simulink model "IntelligentBinPicking"  (R2024a)
settings: Solver=FixedStepAuto  StartTime=0.0  StopTime=200  FixedStep=0.05  RelTol=1e-3
PreLoadFcn:
  | initRobotModelParam;
model workspace (MAT data in the model file):
  SL_ROS_VariableLengthArrays_MaxSizes.CommonInfo.ArrayTruncateAction = 'EmitWarning'
  SL_ROS_VariableLengthArrays_MaxSizes.MsgTypeMap = containers.Map
  SL_ROS_VariableLengthArrays_MaxSizes.MsgTypeMap.serialization.keys = {'sensor_msgs/Image', 'sensor_msgs/PointCloud2'}
  SL_ROS_VariableLengthArrays_MaxSizes.MsgTypeMap.serialization.values{1}(1).PropertyName = 'Data'
  SL_ROS_VariableLengthArrays_MaxSizes.MsgTypeMap.serialization.values{1}(1).DataType = 'uint8'
  SL_ROS_VariableLengthArrays_MaxSizes.MsgTypeMap.serialization.values{1}(1).MaxLength = 921600
  SL_ROS_VariableLengthArrays_MaxSizes.MsgTypeMap.serialization.values{1}(2).PropertyName = 'Encoding'
  SL_ROS_VariableLengthArrays_MaxSizes.MsgTypeMap.serialization.values{1}(2).DataType = 'uint8'
  SL_ROS_VariableLengthArrays_MaxSizes.MsgTypeMap.serialization.values{1}(2).MaxLength = 128
  SL_ROS_VariableLengthArrays_MaxSizes.MsgTypeMap.serialization.values{2}(1).PropertyName = 'Data'
  SL_ROS_VariableLengthArrays_MaxSizes.MsgTypeMap.serialization.values{2}(1).DataType = 'uint8'
  SL_ROS_VariableLengthArrays_MaxSizes.MsgTypeMap.serialization.values{2}(1).MaxLength = 9830400
  SL_ROS_VariableLengthArrays_MaxSizes.MsgTypeMap.serialization.values{2}(2).PropertyName = 'Fields'
  SL_ROS_VariableLengthArrays_MaxSizes.MsgTypeMap.serialization.values{2}(2).DataType = 'sensor_msgs/PointField'
  SL_ROS_VariableLengthArrays_MaxSizes.MsgTypeMap.serialization.values{2}(2).MaxLength = 16
  SL_ROS_VariableLengthArrays_MaxSizes.MsgTypeMap.serialization.uniformity = 0
  SL_ROS_VariableLengthArrays_MaxSizes.MsgTypeMap.serialization.keyType = 'char'
  SL_ROS_VariableLengthArrays_MaxSizes.MsgTypeMap.serialization.valueType = 'any'
undefined symbols (not defined in the file): binActorRotationSequenceInfo, binActorTranslationSequenceInfo, binCenterPosition, camera_rot, cameraIntrinsics, cx_camera, cy_camera, downSampleForTrajectoryWaypoints, Enable, enumCmd, f, graspRegionTranslation, gray, homePosition, IsAccValid, IsMoving, IsPosValid, isSingleDetection, IsValid, IsVelValid, JointAcc, JointCurrent, JointPos, JointTrajectory, JointVel, maxVisionObjects, Mode, motionPlannerCmdInitValue, motionPlannerResponseInitValue, NumObjects, NumPoints, objectDetectorResponseInitValue, Objects, ObjectTypesID, pickAllOrder, PickAllOrder, PickAndPlaceModes, PickSelectedObjectID, posTargetError, predictionConfidenceScore, RequestID, Reset, RGBCameraTransform, robotCommandInitValue, robotFeedbackInitValue, Sim3dSensor, Status, TargetEETranslation, targetEnv, TaskPlannerSampleTime, Time, TooltipTransform, ur5e
libraries: sim3dlib x13, robotlib x6, robotmaniplib x4, robotcorelib x1, robotsim3dlib x1, sim3dcameralib x1
(part 1 of 2)
settings Model: Creator=gjohn  LastModifiedBy=adityas
settings DebuggingCC: SubsystemReferenceDiagnosticForUnitTest=warning
settings RTWCC: GPUComputeCapability=3.5

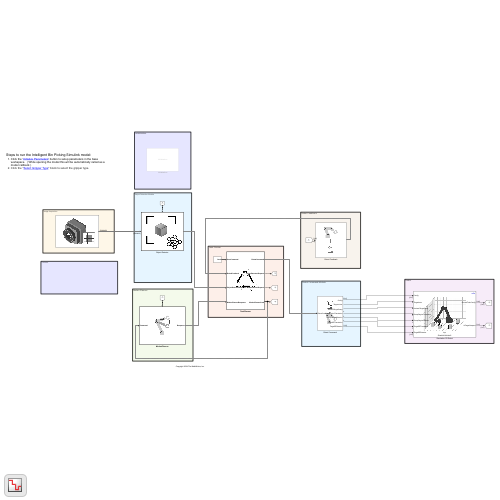
[thumbnail: Simulink's stored preview of the top-level diagram]
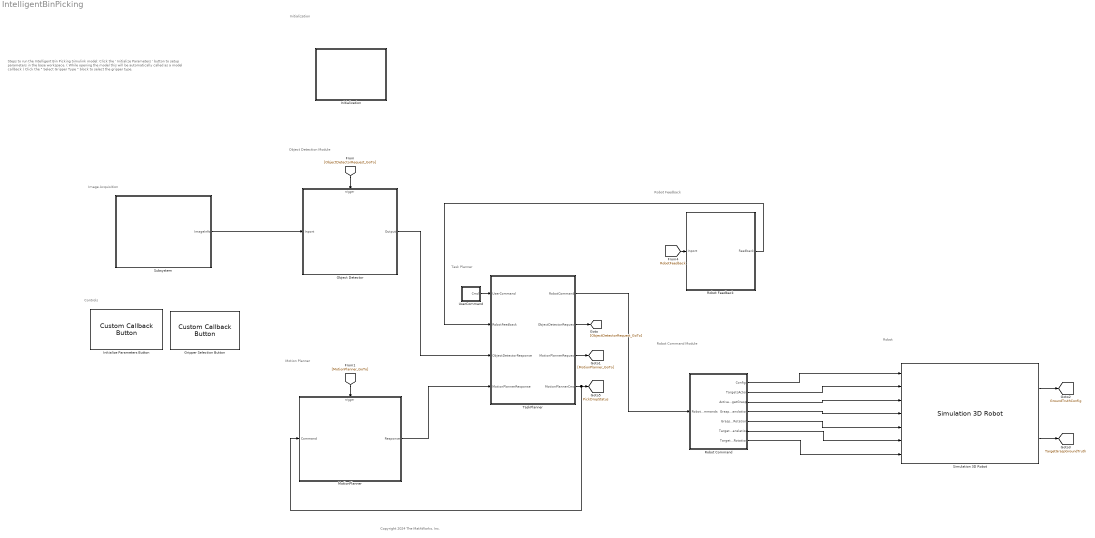
== system IntelligentBinPicking ==
  note: Steps to run the Intelligent Bin Picking Simulink model:
      | Click the ' Initialize Parameters ' button to setup parameters in the base workspace. ( While opening the model this will be automatically called as a model callback )
      | Click the " Select Gripper Type " block to select the gripper type.
  note: Task Planner
  note: Motion Planner
  note: Robot Command Module
  note: Robot Feedback
  note: Object Detection Module
  note: Controls
  note: Copyright 2024 The MathWorks, Inc.
  note: Initialization
  note: Image Acquisition
  note: Robot
  Gripper Selection Button : CustomCallbackButton  Configuration="{\"components\":[{\"name\":\"BackgroundImageComponent\",\"settings\":{\"image\":{\"size\":[0,0],\"src\":\"default\",\"srcOrientation\":\"Right\"},\"position\":[0,0,1,1]}},{\"name\":\"ButtonStateComponent\",\"settings\":{\"buttonType\":\"momentary\",\"clickFcn\":\"getGripperType;\\nfprintf('Loading Robot Model and Parameters...');\\nfprintf('\\\\n');\\nclear rbt ur5e;\\nrbt = loadrobot('universalUR5e','DataFormat','row');\\nur5e = exampleHelperAddGripper(rbt,gripperType);\\n\\ndisp(\\\"Setup complete for Robot hardware\\\");\\n\",\"onValue\":1,\"position\":[0,0,1,1],\"pressDelay\":\"500\",\"pressFcn\":\"\",\"repeatInterval\":\"0\",\"states\":[{\"horizontalAlignment\":\"center\",\"image\":{\"position\":[0,0,1,1],\"size\":[1,1],\"src\":\"default\",\"srcOrientation\":\"Right\"},\"label\":{\"color\":[0.011764705882352941,0.011764705882352941,0.011764705882352941],\"icon\":{\"size\":[0,0],\"src\":\"default\",\"srcOrientation\":\"Right\"},\"iconPlacement\":\"left\",\"opacity\":1,\"show\":true,\"text\":{\"content\":\"Select Gripper Type\",\"font\":\"Helvetica\",\"fontSize\":9.600000000000001}},\"labelOffset\":[0,0],\"verticalAlignment\":\"middle\"},{\"horizontalAlignment\":\"center\",\"image\":{\"position\":[0,0,1,1],\"size\":[1,1],\"src\":\"default\",\"srcOrientation\":\"Right\"},\"label\":{\"color\":[0.011764705882352941,0.011764705882352941,0.011764705882352941],\"icon\":{\"size\":[0,0],\"src\":\"default\",\"srcOrientation\":\"Right\"},\"iconPlacement\":\"left\",\"opacity\":1,\"show\":true,\"text\":{\"content\":\"Select Gripper Type\",\"font\":\"Helvetica\",\"fontSize\":9.600000000000001}},\"labelOffset\":[0,0],\"verticalAlignment\":\"middle\"},{\"horizontalAlignment\":\"center\",\"image\":{\"position\":[0,0,1,1],\"size\":[1,1],\"src\":\"default\",\"srcOrientation\":\"Right\"},\"label\":{\"color\":[0.011764705882352941,0.011764705882352941,0.011764705882352941],\"icon\":{\"size\":[0,0],\"src\":\"default\",\"srcOrientation\":\"Right\"},\"iconPlacement\":\"left\",\"opacity\":1,\"show\":true,\"text\":{\"content\":\"Select Gripper Type\",\"font\":\"Helvetica\",\"fontSize\":9.600000000000001}},\"labelOffset\":[0,0],\"verticalAlignment\":\"middle\"},{\"horizontalAlignment\":\"center\",\"image\":{\"position\":[0,0,1,1],\"size\":[1,1],\"src\":\"default\",\"srcOrientation\":\"Right\"},\"label\":{\"color\":[0.011764705882352941,0.011764705882352941,0.011764705882352941],\"icon\":{\"size\":[0,0],\"src\":\"default\",\"srcOrientation\":\"Right\"},\"iconPlacement\":\"left\",\"opacity\":1,\"show\":true,\"text\":{\"content\":\"Select Gripper Type\",\"font\":\"Helvetica\",\"fontSize\":9.600000000000001}},\"labelOffset\":[0,0],\"verticalAlignment\":\"middle\"}]}},{\"name\":\"ForegroundImageComponent\",\"settings\":{\"image\":{\"size\":[0,0],\"src\":\"default\",\"srcOrientation\":\"Right\"},\"isForeground\":1,\"position\":[0,0,1,1]}}],\"settings\":{\"BindingType\":\"standalone\",\"backgroundColor\":[244,244,244,1],\"backgroundOffset\":0,\"backgroundOpacity\":1,\"fixedAspectRatio\":\"off\",\"foregroundColor\":[0.01176470588,0.01176470588,0.01176470588,1],\"migratedFromLegacy\":true,\"useBackgroundColor\":true,\"variant\":\"callback\",\"version\":\"R2023a\"},\"type\":\"Button\"}"  CustomBackgroundColor="{\"color\":[0.6196078431372549,0.8392156862745098,0.9490196078431372],\"show\":true}"
  Initialization : Subsystem  Priority=0
      mask Display: disp(' Initialization ');
  Initialize Parameters Button : CustomCallbackButton  Configuration="{\"components\":[{\"name\":\"BackgroundImageComponent\",\"settings\":{\"image\":{\"size\":[0,0],\"src\":\"default\",\"srcOrientation\":\"Right\"},\"position\":[0,0,1,1]}},{\"name\":\"ButtonStateComponent\",\"settings\":{\"buttonType\":\"momentary\",\"clickFcn\":\"%%\\ninitRobotModelParam;\\ndisp('*******************************************************');\\ndisp('Parameters Initialized')\",\"onValue\":1,\"position\":[0,0,1,1],\"pressDelay\":\"500\",\"pressFcn\":\"\",\"repeatInterval\":\"0\",\"states\":[{\"horizontalAlignment\":\"center\",\"image\":{\"position\":[0,0,1,1],\"size\":[1,1],\"src\":\"default\",\"srcOrientation\":\"Right\"},\"label\":{\"color\":[0,0,0],\"icon\":{\"size\":[0,0],\"src\":\"default\",\"srcOrientation\":\"Right\"},\"iconPlacement\":\"left\",\"opacity\":1,\"show\":true,\"text\":{\"content\":\"Initialize Parameters\",\"font\":\"Helvetica\",\"fontSize\":3.823752}},\"labelOffset\":[0,0],\"verticalAlignment\":\"middle\"},{\"horizontalAlignment\":\"center\",\"image\":{\"position\":[0,0,1,1],\"size\":[1,1],\"src\":\"default\",\"srcOrientation\":\"Right\"},\"label\":{\"color\":[0.01176470588,0.01176470588,0.01176470588,1],\"icon\":{\"size\":[0,0],\"src\":\"default\",\"srcOrientation\":\"Right\"},\"iconPlacement\":\"left\",\"opacity\":1,\"show\":true,\"text\":{\"content\":\"Initialize Parameters\",\"font\":\"Helvetica\",\"fontSize\":3.823752}},\"labelOffset\":[0,0],\"verticalAlignment\":\"middle\"},{\"horizontalAlignment\":\"center\",\"image\":{\"position\":[0,0,1,1],\"size\":[1,1],\"src\":\"default\",\"srcOrientation\":\"Right\"},\"label\":{\"color\":[0.01176470588,0.01176470588,0.01176470588,1],\"icon\":{\"size\":[0,0],\"src\":\"default\",\"srcOrientation\":\"Right\"},\"iconPlacement\":\"left\",\"opacity\":1,\"show\":true,\"text\":{\"content\":\"Initialize Parameters\",\"font\":\"Helvetica\",\"fontSize\":3.823752}},\"labelOffset\":[0,0],\"verticalAlignment\":\"middle\"},{\"horizontalAlignment\":\"center\",\"image\":{\"position\":[0,0,1,1],\"size\":[1,1],\"src\":\"default\",\"srcOrientation\":\"Right\"},\"label\":{\"color\":[0.01176470588,0.01176470588,0.01176470588,1],\"icon\":{\"size\":[0,0],\"src\":\"default\",\"srcOrientation\":\"Right\"},\"iconPlacement\":\"left\",\"opacity\":1,\"show\":true,\"text\":{\"content\":\"Initialize Parameters\",\"font\":\"Helvetica\",\"fontSize\":3.823752}},\"labelOffset\":[0,0],\"verticalAlignment\":\"middle\"}]}},{\"name\":\"ForegroundImageComponent\",\"settings\":{\"image\":{\"size\":[0,0],\"src\":\"default\",\"srcOrientation\":\"Right\"},\"isForeground\":1,\"position\":[0,0,1,1]}}],\"settings\":{\"BindingType\":\"standalone\",\"backgroundColor\":[244,244,244,1],\"backgroundOffset\":0,\"backgroundOpacity\":1,\"fixedAspectRatio\":\"off\",\"foregroundColor\":[0.01176470588,0.01176470588,0.01176470588,1],\"migratedFromLegacy\":true,\"useBackgroundColor\":true,\"variant\":\"callback\",\"version\":\"R2023a\"},\"type\":\"Button\"}"  CustomBackgroundColor="{\"color\":[0.6196078431372549,0.8392156862745098,0.9490196078431372],\"show\":true}"
  MotionPlanner : Subsystem
      mask Display: image('$imagefile'); % Use "Edit Image" on toolstrip to change.
  Object Detector : Subsystem  TreatAsAtomicUnit=on
      mask Display: image('$imagefile'); % Use "Edit Image" on toolstrip to change.
  Robot Command : Subsystem
      mask Display: image('SLToRobotComm.png');
  Robot Feedback : Subsystem
      mask Display: image('$imagefile'); % Use "Edit Image" on toolstrip to change.
  Simulation 3D Robot : robotsim3dlib/Simulation 3D Robot  actorInputType=RigidBodyTree Object  RigidBodyTree=ur5e  ActorName=SimulinkVehicle2  existActorChekBox=off  initialTrans=robotInitialBaseTranslation  initialRot=robotInitialBaseRotation  initialConfig=homePosition  EndEffector=tcp  eeOffsetInpChekBox=on  eeTargetTrans=[0 0 0.015 ]  eeTargetRot=[ 0 0 0 ]  enableRegionGraspChekBox=on  regionGraspInpChekBox=on  eeTargTransDiff=[ 0.2 0.2 0.2 ]  eeTargRotDiff=[ 0 0 0 ]  inpConfEnbVal=on  inpGraspEnbVal=on  inpTransEnbVal=off  outConfEnbVal=on  outGraspEnbVal=on  outTransEnbVal=off  SampleTime=-1  ActorType=SimulinkVehicle  ID=2  aMode=6  ActorTag=SimulinkVehicle2  Mesh=RigidBodyTree
  Subsystem : Subsystem
      mask Display:
      | IconInfoM = sim3dblkssharedicon('sim3dblkscamerasensor', gcb, 'DrawCommands');
      | image(IconInfoM.image);
  TaskPlanner : Subsystem  TreatAsAtomicUnit=on  SystemSampleTime=TaskPlannerSampleTime
      mask Display: image('$imagefile'); % Use "Edit Image" on toolstrip to change.
  UserCommand : Subsystem
  tag scope: GroundTruthConfig=global, PickDropStatus=global, TargetGraspGroundTruth=global
  wires:
  UserCommand/1(Cmd) -> TaskPlanner/1(UserCommand)
  TaskPlanner/2(ObjectDetectorRequest) -> [ObjectDetectorRequest_GoTo]
  [ObjectDetectorRequest_GoTo] -> Object Detector/Trigger
  TaskPlanner/3(MotionPlannerRequest) -> [MotionPlanner_GoTo]
  [MotionPlanner_GoTo] -> MotionPlanner/Trigger
  TaskPlanner/4(MotionPlannerCmd) -> [PickDropStatus], MotionPlanner/1(Command)
  MotionPlanner/1(Response) -> TaskPlanner/4(MotionPlannerResponse)
  Object Detector/1(Output) -> TaskPlanner/3(ObjectDetectorResponse)
  Robot Feedback/1(Feedback) -> TaskPlanner/2(RobotFeedback)
  Simulation 3D Robot/1 -> [GroundTruthConfig]
  Simulation 3D Robot/2 -> [TargetGraspGroundTruth]
  [RobotFeedback] -> Robot Feedback/1(Inport)
  Subsystem/1(ImageInfo) -> Object Detector/1(Inport)
  TaskPlanner/1(RobotCommand) -> Robot Command/1(RobotCommands)
  Robot Command/1(Config) -> Simulation 3D Robot/1
  Robot Command/2(TargetcActor) -> Simulation 3D Robot/2
  Robot Command/3(ActivateTargetGrasp) -> Simulation 3D Robot/3
  Robot Command/4(GraspRegionTranslation) -> Simulation 3D Robot/4
  Robot Command/5(GraspRegionRotation) -> Simulation 3D Robot/5
  Robot Command/6(TargetEETranslation) -> Simulation 3D Robot/6
  Robot Command/7(TargetEERotation) -> Simulation 3D Robot/7

== system IntelligentBinPicking/Initialization ==
  Sim3d Scene Generation : Subsystem
      mask Display:
      | IconInfo = sim3dblkssharedicon('sim3dblksgenericactor',gcb,'DrawCommands');
      | image(IconInfo.image);
  Simulation 3D Scene Configuration : sim3dlib/Simulation 3D Scene Configuration  Priority=0  ProjectFormat=Default Scenes  SceneDesc=Empty scene  ProjectName=S:\41\adityas.BR2024ad.j2628055.GeckIBP\matlab\toolbox\shared\sim3d_projects\automotive_project_windows\UE\WindowsNoEditor\VehicleSimulation.exe  ScenePath=/Game/Maps/HwStrght  EnableOpenDRIVE=off  vehTagList={'BackPlane';'CelingPlane';'Custom';'FrontPlane';'GroundPlane';'LeftPlane';'RightPlane';'Scene Origin';'Sim3dActor1';'Sim3dActor2';'Sim3dActor3';'Sim3dActor4';'Sim3dActor5';'SimulinkVehicle2';'TableStand'}  vehTag=Custom  FreeCameraInitialTranslation=[0.25 1.5 1.0]  FreeCameraDefaultInitialTranslation=[-6, 0, 2]  FreeCameraInitialRotation=[-30, 0, -100]  FreeCameraDefaultInitialRotation=[0, -15, 0]  OpVisEn=off  Ts=0.05  EnableWindow=on  EnableRemoteAccess=off  EnableWeather=on  SunAzimuth=180  SunAltitude=90  EnableGeospatialSun=off  Latitude=0  Longitude=0  Date=2023-01-01  Time=10:30:00  GeoTimeZone=-5.0  SunDaylightSaving=off  wind=-6.0  clouds=0  EnableVolumetricClouds=off  CloudCoverage=50  CloudAltitude=5  fog=0  rain=0  RaindropsEffect=off  SnowDensity=0  EnableGeospatial=off  UseTrueOrigin=off  OriginHeight=200  OriginLatitude=40.744652  OriginLongitude=-73.988864  MapStyle=Aerial  AdditionalAssetIDs=[]  UseAdvancedSunSky=off  SolarTime=11  TimeZone=-5  Day=21  Month=9  Year=2022  UseDaylightSavingTime=on  DSTStartDay=10  DSTStartMonth=3  DSTEndDay=3  DSTEndMonth=11  DSTSwitchHour=2  sensorTag=MainCamera1  sensorId=1  sensorName=MainCamera1  mountLoc=Origin  offsetFlag=off  tmountOffset=[0, 0, 0]  rmountOffset=[0, 0, 0]  HorizontalResolution=1280  VerticalResolution=720  HorizontalFOV=60  mountPoint=[0 0 0]  mountOrientation=[0 0 0]  aMode=5  ID=1  GeoTrigger=Inactive
      settings: LibrarySourceBlock=sl3dlib/Simulation 3D/Simulation 3D Scene Configuration

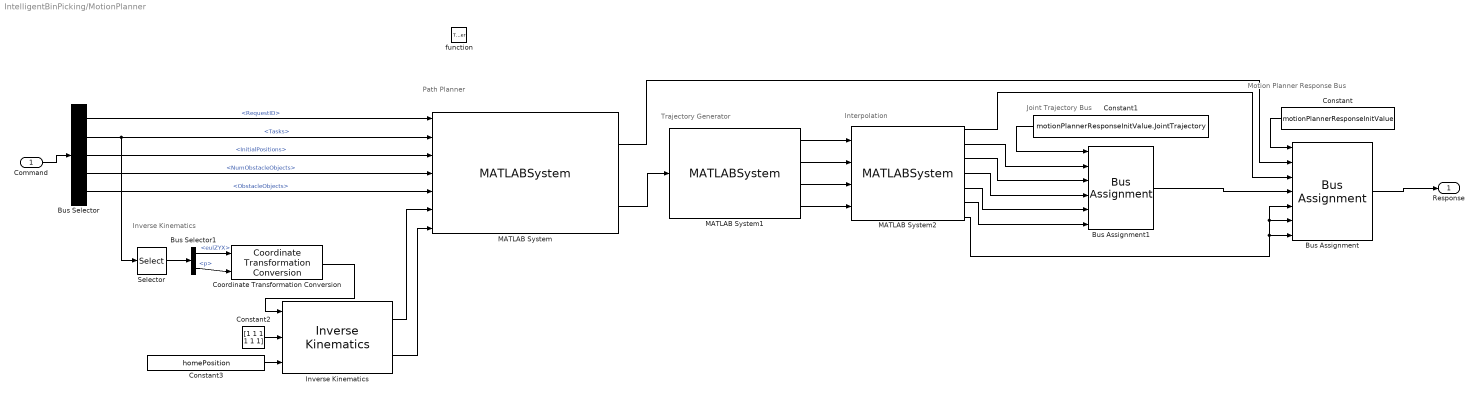
== system IntelligentBinPicking/MotionPlanner ==
  note: Interpolation
  note: Trajectory Generator
  note: Path Planner
  note: Inverse Kinematics
  note: Joint Trajectory Bus
  note: Motion Planner Response Bus
  Command : Inport  OutDataTypeStr=Bus: BUS_motion_planner_cmd
  function : TriggerPort  TriggerType=function-call  VariantControl=Variant  PortDimensions=1
  Bus Assignment : BusAssignment  AssignedSignals=RequestID,Status,JointTrajectory,IsPosValid,IsVelValid,IsAccValid
  Bus Assignment1 : BusAssignment  AssignedSignals=NumPoints,Time,JointPos,JointVel,JointAcc
  Bus Selector : BusSelector  OutputSignals=RequestID,Tasks,InitialPositions,NumObstacleObjects,ObstacleObjects
  Bus Selector1 : BusSelector  OutputSignals=eulZYX,p
  Constant : Constant  Value=motionPlannerResponseInitValue  OutDataTypeStr=Bus: BUS_motion_planner_response
  Constant1 : Constant  Value=motionPlannerResponseInitValue.JointTrajectory  OutDataTypeStr=Bus: BUS_joint_trajectory
  Constant2 : Constant  Value=[1 1 1 1 1 1]
  Constant3 : Constant  Value=homePosition
  Coordinate Transformation Conversion : robotcorelib/Coordinate Transformation Conversion  InputRepresentation=Euler Angles  InputEulerSequence=ZYX  ShowTrVecInputPort=on  OutputRepresentation=Homogeneous Transformation  OutputEulerSequence=ZYX  ShowTrVecOutputPort=on  SimulateUsing=Code generation
  Inverse Kinematics : robotmaniplib/Inverse Kinematics  RigidBodyTree=ur5e  EndEffector=tcp  ShowInfo=on  SolverName=BFGS Gradient Projection  EnforceJointLimits=on  MaxIterations=1500  MaxTime=10  GradientTolerance=1e-7  SolutionTolerance=1e-6  StepTolerance=1e-14  ErrorChangeTolerance=1e-12  UseErrorDamping=on  DampingBias=0.0025  SimulateUsing=Code generation
  MATLAB System : MATLABSystem  System=MotionPlannerCHOMP  BinLength=binLength  BinHeight=binHeight  BinWidth=binWidth  BinRotation=binRotation  BinCenterPosition=binCenterPosition  HomePosition=retractHomePosition  Target=targetEnv  GripperType=gripperType  IsMEXed=off  SimulateUsing=Interpreted execution
      mask Type: MotionPlannerCHOMP
      mask Display:
      | disp('MotionPlannerCHOMP');
      | port_label('input',1,'requestID');
      | port_label('input',2,'tasks');
      | port_label('input',3,'q0');
      | port_label('input',4,'numObstacles');
      | port_label('input',5,'obstacles');
      | port_label('input',6,'configSoln');
      | port_label('input',7,'configSolnInfo');
      | port_label('output',1,'reqID');
      | port_label('output',2,'path');
  MATLAB System1 : MATLABSystem  System=Contopptraj  VelocityLimits=vellimits  AccelLimits=accellimits  NumSamples=50  SimulateUsing=Interpreted execution
      mask Type: Contopptraj
      mask Display:
      | disp('Contopptraj');
      | port_label('input',1,'planPath');
      | port_label('output',1,'q');
      | port_label('output',2,'qd');
      | port_label('output',3,'qdd');
      | port_label('output',4,'t');
  MATLAB System2 : MATLABSystem  System=Interpolation  trajectorySampleTime=1 / 400  MaxNumPoints=maxNumPoints  SimulateUsing=Code generation
      mask Type: Interpolation
      mask Display:
      | disp('Interpolation');
      | port_label('input',1,'q');
      | port_label('input',2,'qd');
      | port_label('input',3,'qdd');
      | port_label('input',4,'t');
      | port_label('output',1,'status');
      | port_label('output',2,'numPoints');
      | port_label('output',3,'time');
      | port_label('output',4,'jointPos');
      | port_label('output',5,'jointVel');
      | port_label('output',6,'jointAcc');
      | port_label('output',7,'isValid');
  Selector : Selector  InputPortWidth=20  IndexOptions=Index vector (dialog)  Indices=1  OutputSizes=1
  Response : Outport  OutDataTypeStr=Bus: BUS_motion_planner_response  InitialOutput=motionPlannerResponseInitValue  VectorParamsAs1DForOutWhenUnconnected=off
  wires:
  Bus Selector1/2 -> Coordinate Transformation Conversion/2  "<p>"
  Bus Selector/3 -> MATLAB System/3  "<InitialPositions>"
  Constant2/1 -> Inverse Kinematics/2
  Selector/1 -> Bus Selector1/1
  Bus Selector/2 -> MATLAB System/2, Selector/1  "<Tasks>"
  Coordinate Transformation Conversion/1 -> Inverse Kinematics/1
  Inverse Kinematics/1 -> MATLAB System/6
  Bus Selector1/1 -> Coordinate Transformation Conversion/1  "<eulZYX>"
  Command/1 -> Bus Selector/1
  Bus Selector/1 -> MATLAB System/1  "<RequestID>"
  MATLAB System2/1 -> Bus Assignment/3
  MATLAB System/1 -> Bus Assignment/2
  MATLAB System2/3 -> Bus Assignment1/3
  MATLAB System2/5 -> Bus Assignment1/5
  MATLAB System2/6 -> Bus Assignment1/6
  Bus Assignment/1 -> Response/1
  Constant1/1 -> Bus Assignment1/1
  MATLAB System2/4 -> Bus Assignment1/4
  MATLAB System2/2 -> Bus Assignment1/2
  Constant/1 -> Bus Assignment/1
  Bus Assignment1/1 -> Bus Assignment/4
  MATLAB System2/7 -> Bus Assignment/5, Bus Assignment/6, Bus Assignment/7
  Bus Selector/4 -> MATLAB System/4  "<NumObstacleObjects>"
  Bus Selector/5 -> MATLAB System/5  "<ObstacleObjects>"
  MATLAB System1/1 -> MATLAB System2/1
  MATLAB System1/2 -> MATLAB System2/2
  MATLAB System1/3 -> MATLAB System2/3
  MATLAB System1/4 -> MATLAB System2/4
  MATLAB System/2 -> MATLAB System1/1
  Inverse Kinematics/2 -> MATLAB System/7
  Constant3/1 -> Inverse Kinematics/3

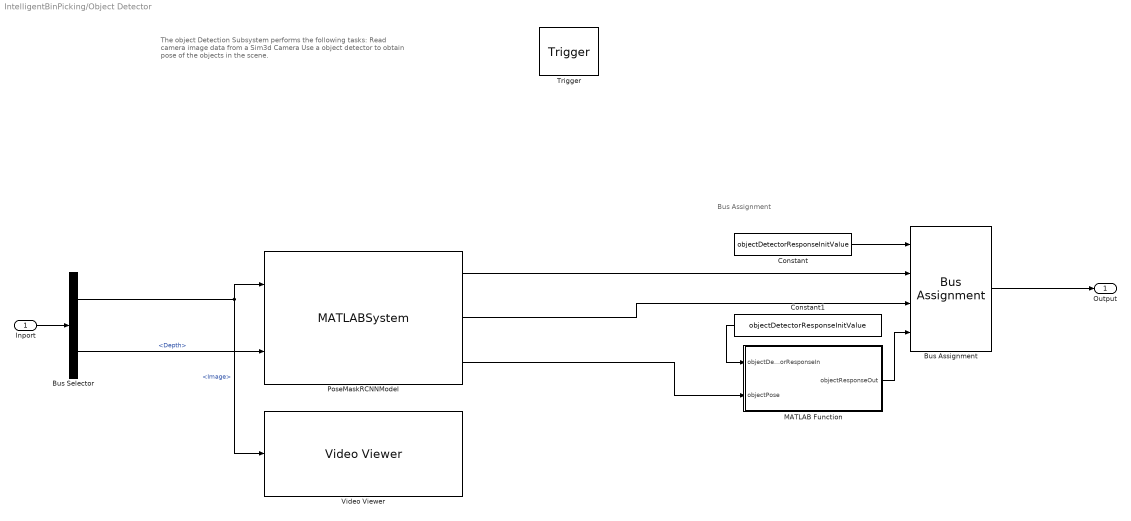
== system IntelligentBinPicking/Object Detector ==
  note: Bus Assignment
  note: The object Detection Subsystem performs the following tasks:
      | Read camera image data from a Sim3d Camera
      | Use a object detector to obtain pose of the objects in the scene.
  Inport : Inport
  Trigger : TriggerPort  TriggerType=function-call  VariantControl=(inherit)
  Bus Assignment : BusAssignment  AssignedSignals=Status,NumObjects,Objects
  Bus Selector : BusSelector  OutputSignals=Image,Depth
  Constant : Constant  Value=objectDetectorResponseInitValue  OutDataTypeStr=Bus: BUS_object_detector_response
  Constant1 : Constant  Value=objectDetectorResponseInitValue  OutDataTypeStr=Bus: BUS_object_detector_response
  MATLAB Function : MATLAB Function  TreatAsAtomicUnit=on
  PoseMaskRCNNModel : MATLABSystem  System=PoseMaskRCNNModel  NetName=resnet50-pvc-parts  MaxDepth=maxDepth  MaxBinDistance=maxBinDistance  BinOrientation=binOrientation  TargetBinaryMask=targetAreaMask  CameraLoc=camera_loc  CameraRot=camera_rot  Intrinsics="cameraIntrinsics( [ 750, 750 ], [ 640, 360 ], [ 720, 1280 ], \"RadialDistortion\", [ 0, 0 ], \"TangentialDistortion\", [ 0, 0 ], \"Skew\", 0 )"  MaxObjectDectection=maxObjectDetection  Threshold=predictionConfidenceScore  RobotOffset=robotInitialBaseTranslation  ExecutionEnvironment=gpu
      mask Type: PoseMaskRCNNModel
      mask Display:
      | disp('PoseMaskRCNNModel');
      | port_label('input',1,'imRGB');
      | port_label('input',2,'imDepth');
      | port_label('output',1,'status');
      | port_label('output',2,'numObjects');
      | port_label('output',3,'objectPose');
  Video Viewer : VideoViewer  colormapValue=gray(256)  FigPos=[345 622 589.333333333333 526]
  Output : Outport
  wires:
  Constant/1 -> Bus Assignment/1
  PoseMaskRCNNModel/1 -> Bus Assignment/2
  PoseMaskRCNNModel/2 -> Bus Assignment/3
  Bus Assignment/1 -> Output/1
  Constant1/1 -> MATLAB Function/1(objectDetectorResponseIn)
  PoseMaskRCNNModel/3 -> MATLAB Function/2(objectPose)
  MATLAB Function/1(objectResponseOut) -> Bus Assignment/4
  Bus Selector/1 -> PoseMaskRCNNModel/1, Video Viewer/1  "<Image>"
  Bus Selector/2 -> PoseMaskRCNNModel/2  "<Depth>"
  Inport/1 -> Bus Selector/1

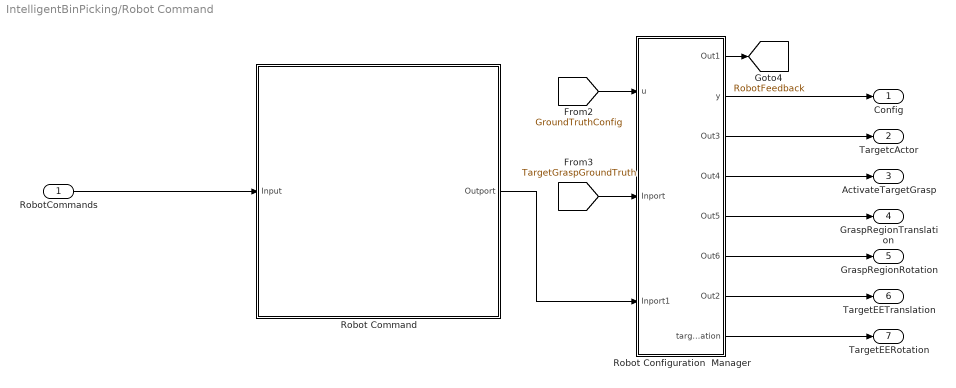
== system IntelligentBinPicking/Robot Command ==
  RobotCommands : Inport
  Robot Command : Subsystem
      mask Display: image('SLToRobotComm.png'); % Use "Edit Image" on toolstrip to change.
  Robot Configuration  Manager : Subsystem  mask{RobotRigidTree=ur5e, ActorTranslationConfig=binActorTranslationSequenceInfo, ActorRotationConfig=binActorRotationSequenceInfo, HomePosition=homePosition, SamplesToConsider=downSampleForTrajectoryWaypoints, GraspRegionTranslation=graspRegionTranslation, TargetEETranslation=TargetEETranslation}
      mask prompts: RobotRigidTree "Robot rigid tree"; ActorTranslationConfig "Actor translation config"; ActorRotationConfig "Actor rotation config"; HomePosition "Robot home position"; SamplesToConsider "Samples to consider"; GraspRegionTranslation "Grasp region translation"; TargetEETranslation "Target-EE Translation"
      mask Display: disp('Config Manager');
  Config : Outport
  TargetcActor : Outport  Port=2
  ActivateTargetGrasp : Outport  Port=3
  GraspRegionTranslation : Outport  Port=4
  GraspRegionRotation : Outport  Port=5
  TargetEETranslation : Outport  Port=6
  TargetEERotation : Outport  Port=7
  tag scope: RobotFeedback=global
  wires:
  Robot Configuration  Manager/1(Out1) -> [RobotFeedback]
  Robot Configuration  Manager/2(y) -> Config/1
  [TargetGraspGroundTruth] -> Robot Configuration  Manager/2(Inport)
  [GroundTruthConfig] -> Robot Configuration  Manager/1(u)
  Robot Configuration  Manager/4(Out4) -> ActivateTargetGrasp/1
  Robot Command/1(Outport) -> Robot Configuration  Manager/3(Inport1)
  Robot Configuration  Manager/5(Out5) -> GraspRegionTranslation/1
  Robot Configuration  Manager/3(Out3) -> TargetcActor/1
  RobotCommands/1 -> Robot Command/1(Input)
  Robot Configuration  Manager/6(Out6) -> GraspRegionRotation/1
  Robot Configuration  Manager/7(Out2) -> TargetEETranslation/1
  Robot Configuration  Manager/8(targetBinActorOrientation) -> TargetEERotation/1

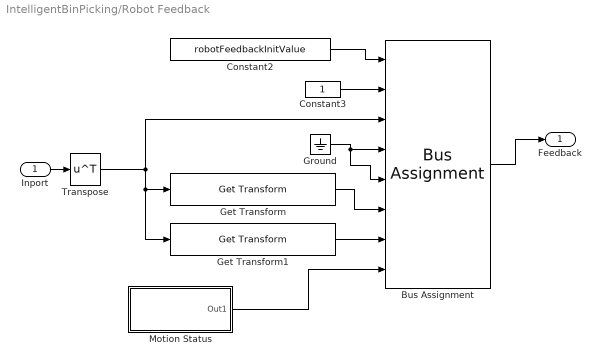
== system IntelligentBinPicking/Robot Feedback ==
  Inport : Inport
  Bus Assignment : BusAssignment  AssignedSignals=IsValid,JointPos,JointVel,JointCurrent,TooltipTransform,RGBCameraTransform,IsMoving
  Constant2 : Constant  Value=robotFeedbackInitValue  OutDataTypeStr=Bus: BUS_robot_feedback
  Constant3 : Constant  OutDataTypeStr=boolean
  Get Transform : robotmaniplib/Get Transform  RigidBodyTree=ur5e  SourceBody=tcp  TargetBody=base_link  SimulateUsing=Interpreted execution
  Get Transform1 : robotmaniplib/Get Transform  RigidBodyTree=ur5e  SourceBody=base_link  TargetBody=base_link  SimulateUsing=Interpreted execution
  Ground : Ground
  Motion Status : Subsystem  Variant=on
  Transpose : Math  Operator=transpose
  Feedback : Outport  OutDataTypeStr=Bus: BUS_robot_feedback  VectorParamsAs1DForOutWhenUnconnected=off
  wires:
  Get Transform1/1 -> Bus Assignment/7
  Constant2/1 -> Bus Assignment/1
  Bus Assignment/1 -> Feedback/1
  Ground/1 -> Bus Assignment/5, Bus Assignment/4
  Get Transform/1 -> Bus Assignment/6
  Constant3/1 -> Bus Assignment/2
  Motion Status/1(Out1) -> Bus Assignment/8
  Transpose/1 -> Bus Assignment/3, Get Transform1/1, Get Transform/1
  Inport/1 -> Transpose/1

== system IntelligentBinPicking/Subsystem ==
  Bus Creator : BusCreator  Inputs=2
  Simulation 3D Camera1 : sim3dcameralib/Simulation 3D Camera  Priority=1  sensorTag=Sim3dSensor�  sensorId=4  sensorName=Sim3dSensor�  vehTagList={'BackPlane';'CelingPlane';'FrontPlane';'GroundPlane';'LeftPlane';'RightPlane';'Scene Origin';'Sim3dActor1';'Sim3dActor2';'SimulinkVehicle2';'TableStand'}  vehTag=Scene Origin  mountLoc=Origin  offsetFlag=on  tmountOffset=camera_loc  extTmount=off  rmountOffset=rad2deg(camera_rot)  extRmount=off  FocalLength=[f, f]  OpticalCenter=[cx_camera, cy_camera]  ImageSize=imageSize  RadialDistortion=[0, 0]  TangentialDistortion=[0, 0]  SensorSkew=0  DepthOutportEnabled=on  SemanticOutportEnabled=off  TransformOutportEnabled=off  SampleTime=-1  mountPoint=[0.48 0 1.15]  mountOrientation=[90 -90 -90]  aMode=3  ID=4
      settings: LibrarySourceBlock=drivingsim3d/Simulation 3D Camera
  ImageInfo : Outport
  wires:
  Simulation 3D Camera1/1 -> Bus Creator/1  "Image"
  Simulation 3D Camera1/2 -> Bus Creator/2  "Depth"
  Bus Creator/1 -> ImageInfo/1

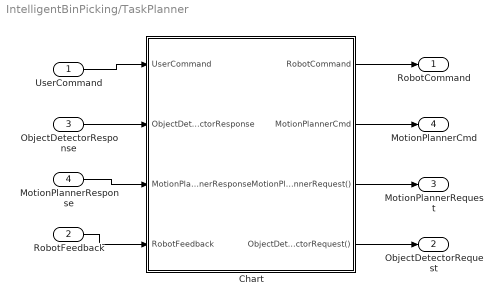
== system IntelligentBinPicking/TaskPlanner ==
  UserCommand : Inport
  RobotFeedback : Inport  Port=2  OutDataTypeStr=Bus: BUS_robot_feedback
  ObjectDetectorResponse : Inport  Port=3  OutDataTypeStr=Bus: BUS_object_detector_response
  MotionPlannerResponse : Inport  Port=4
  Chart : Stateflow chart  TreatAsAtomicUnit=on
  RobotCommand : Outport  OutDataTypeStr=Bus: BUS_robot_command  VectorParamsAs1DForOutWhenUnconnected=off
  ObjectDetectorRequest : Outport  Port=2  VectorParamsAs1DForOutWhenUnconnected=off
  MotionPlannerRequest : Outport  Port=3  VectorParamsAs1DForOutWhenUnconnected=off
  MotionPlannerCmd : Outport  Port=4  OutDataTypeStr=Bus: BUS_motion_planner_cmd  VectorParamsAs1DForOutWhenUnconnected=off
  wires:
  Chart/3(MotionPlannerRequest()) -> MotionPlannerRequest/1
  Chart/2(MotionPlannerCmd) -> MotionPlannerCmd/1
  MotionPlannerResponse/1 -> Chart/3(MotionPlannerResponse)
  Chart/4(ObjectDetectorRequest()) -> ObjectDetectorRequest/1
  ObjectDetectorResponse/1 -> Chart/2(ObjectDetectorResponse)
  Chart/1(RobotCommand) -> RobotCommand/1
  UserCommand/1 -> Chart/1(UserCommand)
  RobotFeedback/1 -> Chart/4(RobotFeedback)

== system IntelligentBinPicking/UserCommand ==
  Bus Assignment : BusAssignment  AssignedSignals=Mode,PickSelectedObjectID,PickAllOrder,Enable,Reset
  Bus_0 : Constant  Value=0  OutDataTypeStr=Bus: BUS_user_command
  Enable : Constant  OutDataTypeStr=boolean
  Mode : Constant  Value=PickAndPlaceModes.PickAll  OutDataTypeStr=Enum: PickAndPlaceModes
  ObjectToPick : Constant  Value=ObjectTypesID.X
  PickAllOrder : Constant  Value=pickAllOrder
  Reset : Constant  Value=0  OutDataTypeStr=boolean
  Cmd : Outport  OutDataTypeStr=Bus: BUS_user_command  VectorParamsAs1DForOutWhenUnconnected=off
  wires:
  Bus_0/1 -> Bus Assignment/1
  Bus Assignment/1 -> Cmd/1
  ObjectToPick/1 -> Bus Assignment/3
  Enable/1 -> Bus Assignment/5
  Reset/1 -> Bus Assignment/6
  Mode/1 -> Bus Assignment/2
  PickAllOrder/1 -> Bus Assignment/4

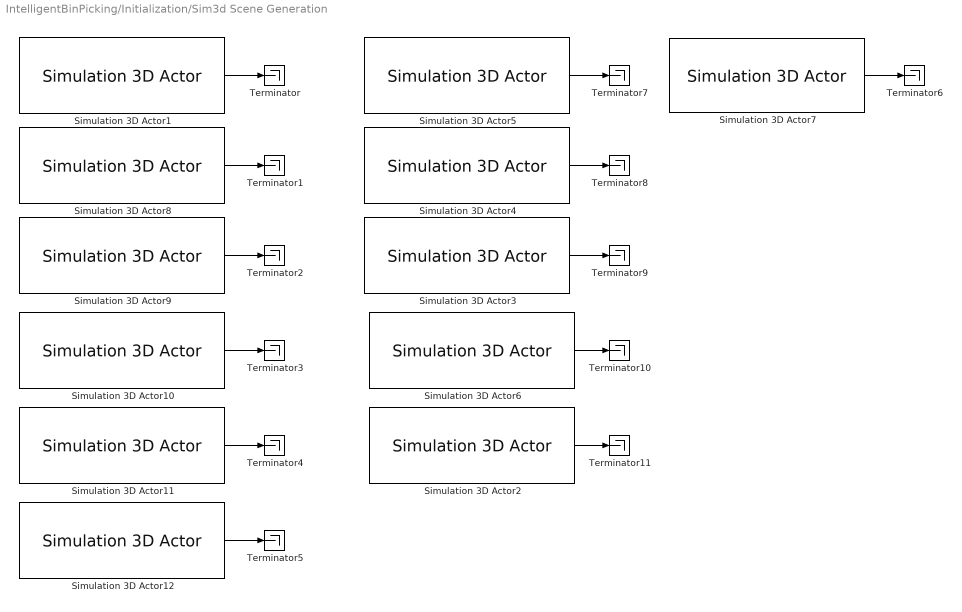
== system IntelligentBinPicking/Initialization/Sim3d Scene Generation ==
  Simulation 3D Actor1 : sim3dlib/Simulation 3D Actor  ActorName=GroundPlane  ParentName=Scene Origin  Operation=Create at setup  InitScriptText=|  SampleTime=-1  Translation=single([0 0 0])  Rotation=single([0 0 0])  Scale=single([1 1 1])  aMode=5  ActorTag=GroundPlane  ActorType=Sim3dActor  ID=C
      | Actor.createShape('box', [3 3 0.05]);
      | Actor.Color=[0.1 0.1 0.1];
      | Actor.Translation=[0 0 0];
      | Actor.Mobility=sim3d.utils.MobilityTypes.Movable;
      | Actor.ConstantAttributes=false;
      settings: LibrarySourceBlock=sl3dlib/Simulation 3D/Simulation 3D Actor
  Simulation 3D Actor10 : sim3dlib/Simulation 3D Actor  ActorName=Sim3dActor3  ParentName=Scene Origin  Operation=Create at setup  InitScriptText=|  SampleTime=-1  Translation=single([0 0 0])  Rotation=single([0 0 0])  Scale=single([1 1 1])  aMode=5  ActorTag=Sim3dActor3  ActorType=Sim3dActor  ID=3
      | %Guider
      | Actor.createShape('box', [0.0050, 0.2000, 0.0050]);
      | Actor.Translation=[0.05 -0.49 0.58];
      | Actor.Rotation=[0 pi/2 pi/2];
      | Actor.Shadows = 0;
      | Actor.Metallic = 0.70;
      | Actor.Color =[0.6824,0.4706,0.4667];
      | Actor.PreciseContacts=true;
      | Actor.Shininess=0.30;
      | Actor.Mobility=sim3d.utils.MobilityTypes.Movable;
      | Actor.ConstantAttributes=false;
      | Actor.Hidden=true;
      settings: LibrarySourceBlock=sl3dlib/Simulation 3D/Simulation 3D Actor
  Simulation 3D Actor11 : sim3dlib/Simulation 3D Actor  ActorName=Sim3dActor4  ParentName=Scene Origin  Operation=Create at setup  InitScriptText=|  SampleTime=-1  Translation=single([0 0 0])  Rotation=single([0 0 0])  Scale=single([1 1 1])  aMode=5  ActorTag=Sim3dActor4  ActorType=Sim3dActor  ID=4
      | %Guider
      | Actor.createShape('box', [0.0050, 0.2000, 0.0050]);
      | Actor.Translation=[0.05 -0.9 0.58];
      | Actor.Rotation=[0 pi/2 pi/2];
      | Actor.Shadows = 0;
      | Actor.Metallic = 0.70;
      | Actor.Color =[0.6824,0.4706,0.4667];
      | Actor.PreciseContacts=true;
      | Actor.Shininess=0.30;
      | Actor.Mobility=sim3d.utils.MobilityTypes.Movable;
      | Actor.ConstantAttributes=false;
      | Actor.Hidden=true;
      settings: LibrarySourceBlock=sl3dlib/Simulation 3D/Simulation 3D Actor
  Simulation 3D Actor12 : sim3dlib/Simulation 3D Actor  ActorName=Sim3dActor5  ParentName=Scene Origin  Operation=Create at setup  InitScriptText=|  SampleTime=-1  Translation=single([0 0 0])  Rotation=single([0 0 0])  Scale=single([1 1 1])  aMode=5  ActorTag=Sim3dActor5  ActorType=Sim3dActor  ID=5
      | %Guider
      | Actor.createShape('box', [0.0050, 0.2000, 0.0050]);
      | Actor.Translation=[0.05 0.5 0.56];
      | Actor.Rotation=[0 pi/2 pi/2];
      | Actor.Shadows = 0;
      | Actor.Metallic = 0.70;
      | Actor.Color =[0.6824,0.4706,0.4667];
      | Actor.PreciseContacts=true;
      | Actor.Shininess=0.30;
      | Actor.Mobility=sim3d.utils.MobilityTypes.Movable;
      | Actor.ConstantAttributes=false;
      | Actor.Hidden=true;
      settings: LibrarySourceBlock=sl3dlib/Simulation 3D/Simulation 3D Actor
  Simulation 3D Actor2 : sim3dlib/Simulation 3D Actor  ActorName=RightPlane  ParentName=Scene Origin  Operation=Create at setup  InitScriptText=|  SampleTime=-1  Translation=single([0 0 0])  Rotation=single([0 0 0])  Scale=single([1 1 1])  aMode=5  ActorTag=RightPlane  ActorType=Sim3dActor  ID=C
      | Actor.createShape('box', [3 3 0.05]);
      | Actor.Color=[0.1 0.1 0.1];
      | Actor.Translation=[0 1.5 0.924];
      | Actor.Rotation=[pi/2 0 0];
      | Actor.Scale=[1,0.635,1];
      | Actor.Mobility=sim3d.utils.MobilityTypes.Movable;
      | Actor.ConstantAttributes=false;
      | Actor.Collisions=false;
      settings: LibrarySourceBlock=sl3dlib/Simulation 3D/Simulation 3D Actor
  Simulation 3D Actor3 : sim3dlib/Simulation 3D Actor  ActorName=FrontPlane  ParentName=Scene Origin  Operation=Create at setup  InitScriptText=|  SampleTime=-1  Translation=single([0 0 0])  Rotation=single([0 0 0])  Scale=single([1 1 1])  aMode=5  ActorTag=FrontPlane  ActorType=Sim3dActor  ID=C
      | Actor.createShape('box', [3 3 0.05]);
      | Actor.Color=[0.1 0.1 0.1];
      | Actor.Translation=[-1.5 0 0.924];
      | Actor.Scale=[0.635,1,1];
      | Actor.Rotation=[0 pi/2 0];
      | Actor.Mobility=sim3d.utils.MobilityTypes.Movable;
      | Actor.ConstantAttributes=false;
      | Actor.Collisions=false;
      settings: LibrarySourceBlock=sl3dlib/Simulation 3D/Simulation 3D Actor
  Simulation 3D Actor4 : sim3dlib/Simulation 3D Actor  ActorName=BackPlane  ParentName=Scene Origin  Operation=Create at setup  InitScriptText=|  SampleTime=-1  Translation=single([0 0 0])  Rotation=single([0 0 0])  Scale=single([1 1 1])  aMode=5  ActorTag=BackPlane  ActorType=Sim3dActor  ID=C
      | Actor.createShape('box', [3 3 0.05]);
      | Actor.Color=[0.1 0.1 0.1];
      | Actor.Translation=[1.5 0 0.924];
      | Actor.Scale=[0.635 1 1];
      | Actor.Rotation=[0 pi/2 0];
      | Actor.Mobility=sim3d.utils.MobilityTypes.Movable;
      | Actor.ConstantAttributes=false;
      | Actor.Collisions=false;
      settings: LibrarySourceBlock=sl3dlib/Simulation 3D/Simulation 3D Actor
  Simulation 3D Actor5 : sim3dlib/Simulation 3D Actor  ActorName=CelingPlane  ParentName=Scene Origin  Operation=Create at setup  InitScriptText=|  SampleTime=-1  Translation=single([0 0 0])  Rotation=single([0 0 0])  Scale=single([1 1 1])  aMode=5  ActorTag=CelingPlane  ActorType=Sim3dActor  ID=C
      | Actor.createShape('box', [3 3 0.05]);
      | Actor.Color=[0.1 0.1 0.1];
      | Actor.Translation=[0 0 1.85];
      | Actor.Mobility=sim3d.utils.MobilityTypes.Movable;
      | Actor.ConstantAttributes=false;
      | Actor.Collisions=false;
      | Actor.Shadows= true;
      | 
      | lightactor = sim3d.Light('ActorName','light1');
      | lightactor.LightType = 'RectLight';
      | lightactor.SourceWidth = 0.58;
      | lightactor.SourceHeight = 0.40;
      | lightactor.Intensity=3000;
      | lightactor.Rotation=[0 -pi/2 0];
      | lightactor.Translation =[0.48+0.35,0,0];
      | World.add(lightactor,Actor);
      settings: LibrarySourceBlock=sl3dlib/Simulation 3D/Simulation 3D Actor
  Simulation 3D Actor6 : sim3dlib/Simulation 3D Actor  ActorName=LeftPlane  ParentName=Scene Origin  Operation=Create at setup  InitScriptText=|  SampleTime=-1  Translation=single([0 0 0])  Rotation=single([0 0 0])  Scale=single([1 1 1])  aMode=5  ActorTag=LeftPlane  ActorType=Sim3dActor  ID=C
      | Actor.createShape('box', [3 3 0.05]);
      | Actor.Color=[0.1 0.1 0.1];
      | Actor.Translation=[0 -1.5 0.924];
      | Actor.Rotation=[pi/2 0 0];
      | Actor.Scale=[1,0.635,1];
      | Actor.Mobility=sim3d.utils.MobilityTypes.Movable;
      | Actor.ConstantAttributes=false;
      | Actor.Collisions=false;
      settings: LibrarySourceBlock=sl3dlib/Simulation 3D/Simulation 3D Actor
  Simulation 3D Actor7 : sim3dlib/Simulation 3D Actor  ActorName=TableStand  ParentName=Scene Origin  Operation=Create at setup  InitScriptText=|  SampleTime=-1  Translation=single([0 0 0])  Rotation=single([0 0 0])  Scale=single([1 1 1])  aMode=5  ActorTag=TableStand  ActorType=Sim3dActor  ID=C
      | load("generateParam.mat");
      | fileName = fullfile(projDir,"Perception","meshes","binPickingStand_scaled.stl");
      | Stand = sim3d.Actor('ActorName', 'Stand');
      | Stand.load(fileName, [1 1 1]);
      | Stand.Rotation = single([0 0 0]);
      | Stand.Translation = single([0 0 0.001]*[1 0 0; 0 -1 0; 0 0 1]);
      | Stand.CoordinateSystem ='MATLAB';
      | Stand.Color =[0.6078,0.5569,0.6275];
      | Stand.Collisions=false;
      | Stand.Shadows = 0;
      | World.add(Stand, Actor);
      | 
      | fileName2 = fullfile(projDir,"Perception","meshes","Bin_STL_Scaled.stl");
      | Tray = sim3d.Actor('ActorName', 'Tray');
      | Tray.load(fileName2, [1 1 0.35]);
      | Tray.Rotation =single([0 0 pi/2]*[1 0 0; 0 -1 0; 0 0 -1]);
      | Tray.Translation = single([0.48 0 0.55]*[1 0 0; 0 -1 0; 0 0 1]);
      | Tray.CoordinateSystem ='MATLAB';
      | Tray.Metallic = 0.70;
      | Tray.Color =[0.2784,0.2667,0.6824];
      | Tray.PreciseContacts=true;
      | Tray.Shininess=0.30;
      | Tray.Shadows = 0;
      | World.add(Tray, Actor);
      | 
      | fileName = fullfile(projDir,"Perception","meshes","table_solid_scaled.stl");
      | Table = sim3d.Actor('ActorName', 'Table');
      | Table.load(fileName, [1 1 1]);
      | Table.Rotation = single([0 0 0]);
      | Table.Translation = single([0.15 0.68 0.40]*[1 0 0; 0 -1 0; 0 0 1]);
      | Table.CoordinateSystem ='MATLAB';
      | Table.Color =[0.6824,0.4706,0.4667];
      | Table.Shadows = 0;
      | Table.Friction= 1;
      | Table.Restitution = 0.15;
      | World.add(Table, Actor);
      | 
      | Table2 = sim3d.Actor('ActorName', 'Table2');
      | Table2.load(fileName, [1 1 1]);
      | Table2.Rotation = single([0 0 0]);
      | Table2.Translation = single([0.15 -0.68 0.40]*[1 0 0; 0 -1 0; 0 0 1]);
      | Table2.CoordinateSystem ='MATLAB';
      | Table2.Color =[0.6824,0.4706,0.4667];
      | Table2.Shadows = 0;
      | Table2.Friction= 1.0;
      | Table2.Restitution = 0.1;
      | World.add(Table2, Actor);
      | 
      | 
      | %Parts
      | for i = 1:param.numInstEachObj*numel(param.model_files)
      |     inst_label = sim3d.utils.SemanticType(param.pose_list(i).instance_label);
      |     aname = sprintf("binActor%d", i);
      |     model = sim3d.Actor('ActorName', aname, ...
      |         'ActorClassId', inst_label);
      |     model.load(param.pose_list(i).model_path, [1 1 1] * 1.1);
      |     model.Mobility = sim3d.utils.MobilityTypes.Movable;
      |     model.ConstantAttributes=false;
      |     model.Gravity = true; 
      |     model.Physics = true;
      |     model.Shadows = true;
      |     model.Translation = param.pose_list(i).loc;
      |     model.Rotation = param.pose_list(i).rot;
      |     model.Shininess = param.Shininess;
      |     model.Color = param.Color;
      |     model.Metallic = param.Metallic;
      |     model.Flat = param.Flat;
      |     model.Mass =0.5;
      |     World.add(model, Actor);
      | end
      settings: LibrarySourceBlock=sl3dlib/Simulation 3D/Simulation 3D Actor
  Simulation 3D Actor8 : sim3dlib/Simulation 3D Actor  ActorName=Sim3dActor1  ParentName=Scene Origin  Operation=Create at setup  InitScriptText=|  SampleTime=-1  Translation=single([0 0 0])  Rotation=single([0 0 0])  Scale=single([1 1 1])  aMode=5  ActorTag=Sim3dActor1  ActorType=Sim3dActor  ID=1
      | Actor.createShape('box', [0.4*0.5*0.1 0.5 0.05*0.1]);
      | Actor.Translation=[0.17 -0.69 0.55];
      | Actor.Rotation=[0 pi/2 0];
      | Actor.Shadows = 0;
      | Actor.Metallic = 0.70;
      | Actor.Color =[0.6824,0.4706,0.4667];
      | Actor.PreciseContacts=true;
      | Actor.Shininess=0.30;
      | Actor.Mobility=sim3d.utils.MobilityTypes.Movable;
      | Actor.ConstantAttributes=false;
      settings: LibrarySourceBlock=sl3dlib/Simulation 3D/Simulation 3D Actor
  Simulation 3D Actor9 : sim3dlib/Simulation 3D Actor  ActorName=Sim3dActor2  ParentName=Scene Origin  Operation=Create at setup  InitScriptText=|  SampleTime=-1  Translation=single([0 0 0])  Rotation=single([0 0 0])  Scale=single([1 1 1])  aMode=5  ActorTag=Sim3dActor2  ActorType=Sim3dActor  ID=2
      | Actor.createShape('box', [0.4*0.5*0.1 0.5 0.05*0.1]);
      | Actor.Translation=[0.17 0.69 0.55];
      | Actor.Rotation=[0 pi/2 0];
      | Actor.Shadows = 0;
      | Actor.Metallic = 0.70;
      | Actor.Color =[0.6824,0.4706,0.4667];
      | Actor.PreciseContacts=true;
      | Actor.Shininess=0.30;
      | Actor.Mobility=sim3d.utils.MobilityTypes.Movable;
      | Actor.ConstantAttributes=false;
      settings: LibrarySourceBlock=sl3dlib/Simulation 3D/Simulation 3D Actor
  Terminator{,1..11} (12 alike) : Terminator
  wires:
  Simulation 3D Actor2/1 -> Terminator11/1
  Simulation 3D Actor1/1 -> Terminator/1
  Simulation 3D Actor3/1 -> Terminator9/1
  Simulation 3D Actor7/1 -> Terminator6/1
  Simulation 3D Actor6/1 -> Terminator10/1
  Simulation 3D Actor4/1 -> Terminator8/1
  Simulation 3D Actor5/1 -> Terminator7/1
  Simulation 3D Actor8/1 -> Terminator1/1
  Simulation 3D Actor9/1 -> Terminator2/1
  Simulation 3D Actor10/1 -> Terminator3/1
  Simulation 3D Actor11/1 -> Terminator4/1
  Simulation 3D Actor12/1 -> Terminator5/1

== system IntelligentBinPicking/Robot Command/Robot Command ==
  Input : Inport
  Bus Creator : BusCreator  Inputs=9
  Bus Selector : BusSelector  OutputSignals=ProcessCommand
  Robot Command Subsystem : Subsystem  TreatAsAtomicUnit=on
  Outport : Outport
  wires:
  Robot Command Subsystem/6(FollowHomePositionWaypoint) -> Bus Creator/6  "FollowHomePositionWaypoint"
  Bus Selector/1 -> Robot Command Subsystem/Enable, Bus Creator/7  "<ProcessCommand>"
  Robot Command Subsystem/5(SendJointTrajectorySignal) -> Bus Creator/5  "SendJointTrajectorySignal"
  Robot Command Subsystem/4(FollowTrajectoryWaypoints) -> Bus Creator/4  "FollowTrajectoryWaypoints"
  Robot Command Subsystem/3(DeactivateVacuumValue) -> Bus Creator/3  "DeactivateVacuumValue"
  Input/1 -> Robot Command Subsystem/1(Input), Bus Selector/1
  Robot Command Subsystem/2(ActivateVacuumSignal) -> Bus Creator/2  "ActivateVacuumSignal"
  Robot Command Subsystem/1(ActivateVacuumValue) -> Bus Creator/1  "ActivateVacuumValue"
  Robot Command Subsystem/7(DeactivateVacuumSignal) -> Bus Creator/8  "DeactivateVacuumSignal"
  Robot Command Subsystem/8(SendHomePositionSignal) -> Bus Creator/9  "SendHomePositionSignal"
  Bus Creator/1 -> Outport/1

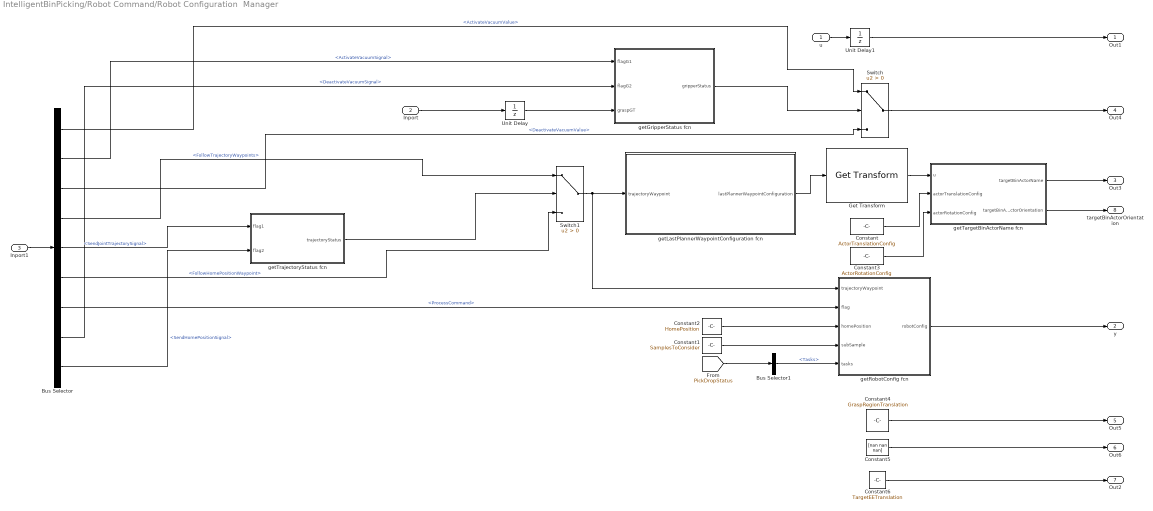
== system IntelligentBinPicking/Robot Command/Robot Configuration  Manager ==
  u : Inport
  Inport : Inport  Port=2
  Inport1 : Inport  Port=3
  Bus Selector : BusSelector  OutputSignals=ActivateVacuumValue,ActivateVacuumSignal,DeactivateVacuumValue,FollowTrajectoryWaypoints,SendJointTrajectorySignal,FollowHomePositionWaypoint,ProcessCommand,DeactivateVacuumSignal,SendHomePositionSignal
  Bus Selector1 : BusSelector  OutputSignals=Tasks
  Constant : Constant  Value=ActorTranslationConfig
  Constant1 : Constant  Value=SamplesToConsider
  Constant2 : Constant  Value=HomePosition
  Constant3 : Constant  Value=ActorRotationConfig
  Constant4 : Constant  Value=GraspRegionTranslation
  Constant5 : Constant  Value=[nan nan nan]
  Constant6 : Constant  Value=TargetEETranslation
  Get Transform : robotmaniplib/Get Transform  RigidBodyTree=RobotRigidTree  SourceBody=tcp  TargetBody=base_link  SimulateUsing=Interpreted execution
  Switch : Switch  Criteria=u2 > Threshold  SaturateOnIntegerOverflow=off  InputSameDT=off
  Switch1 : Switch  Criteria=u2 > Threshold  AllowDiffInputSizes=on  SaturateOnIntegerOverflow=off  InputSameDT=off
  Unit Delay : UnitDelay  InitialCondition=false  SampleTime=-1  HasFrameUpgradeWarning=on
  Unit Delay1 : UnitDelay  InitialCondition=homePosition  SampleTime=-1  HasFrameUpgradeWarning=on
  getGripperStatus fcn : MATLAB Function  TreatAsAtomicUnit=on
  getLastPlannerWaypointConfiguration fcn : MATLAB Function  TreatAsAtomicUnit=on
  getRobotConfig fcn : MATLAB Function  TreatAsAtomicUnit=on
  getTargetBinActorName fcn : MATLAB Function  TreatAsAtomicUnit=on
  getTrajectoryStatus fcn : MATLAB Function  TreatAsAtomicUnit=on
  Out1 : Outport
  y : Outport  Port=2
  Out3 : Outport  Port=3
  Out4 : Outport  Port=4
  Out5 : Outport  Port=5
  Out6 : Outport  Port=6
  Out2 : Outport  Port=7
  targetBinActorOrientation : Outport  Port=8
  wires:
  Constant4/1 -> Out5/1
  Constant5/1 -> Out6/1
  u/1 -> Unit Delay1/1
  Inport/1 -> Unit Delay/1
  Inport1/1 -> Bus Selector/1
  Unit Delay1/1 -> Out1/1
  Unit Delay/1 -> getGripperStatus fcn/3(graspGT)
  Bus Selector/1 -> Switch/1  "<ActivateVacuumValue>"
  Bus Selector/2 -> getGripperStatus fcn/1(flagG1)  "<ActivateVacuumSignal>"
  Bus Selector/3 -> Switch/3  "<DeactivateVacuumValue>"
  Bus Selector/4 -> Switch1/1  "<FollowTrajectoryWaypoints>"
  getTargetBinActorName fcn/1(targetBinActorName) -> Out3/1
  Bus Selector/5 -> getTrajectoryStatus fcn/1(flag1)  "<SendJointTrajectorySignal>"
  Bus Selector/6 -> Switch1/3  "<FollowHomePositionWaypoint>"
  Bus Selector/7 -> getRobotConfig fcn/2(flag)  "<ProcessCommand>"
  Bus Selector/8 -> getGripperStatus fcn/2(flagG2)  "<DeactivateVacuumSignal>"
  Bus Selector/9 -> getTrajectoryStatus fcn/2(flag2)  "<SendHomePositionSignal>"
  getGripperStatus fcn/1(gripperStatus) -> Switch/2
  getTrajectoryStatus fcn/1(trajectoryStatus) -> Switch1/2
  Switch/1 -> Out4/1
  Switch1/1 -> getRobotConfig fcn/1(trajectoryWaypoint), getLastPlannerWaypointConfiguration fcn/1(trajectoryWaypoint)
  getLastPlannerWaypointConfiguration fcn/1(lastPlannerWaypointConfiguration) -> Get Transform/1
  getRobotConfig fcn/1(robotConfig) -> y/1
  Get Transform/1 -> getTargetBinActorName fcn/1(u)
  Constant/1 -> getTargetBinActorName fcn/2(actorTranslationConfig)
  Constant2/1 -> getRobotConfig fcn/3(homePosition)
  Constant1/1 -> getRobotConfig fcn/4(subSample)
  [PickDropStatus] -> Bus Selector1/1
  Bus Selector1/1 -> getRobotConfig fcn/5(tasks)  "<Tasks>"
  getTargetBinActorName fcn/2(targetBinActorOrientation) -> targetBinActorOrientation/1
  Constant3/1 -> getTargetBinActorName fcn/3(actorRotationConfig)
  Constant6/1 -> Out2/1

== system IntelligentBinPicking/Robot Feedback/Motion Status ==
  note: 1) Add Subsystem or Model blocks as valid variant choices.
      | 2) You cannot connect blocks at this level. At simulation, connectivity is automatically
      | determined, based on the active variant and port name matching.
  Gazebo : Subsystem  VariantControl=targetEnv == TargetEnvs.Gazebo
  Hardware : Subsystem  VariantControl=targetEnv == TargetEnvs.Hardware
  Sim3d : Subsystem  VariantControl=targetEnv == TargetEnvs.Sim3d
  Out1 : Outport

== system IntelligentBinPicking/TaskPlanner/Chart/Stop ==
  f : TriggerPort  TriggerType=function-call  VariantControl=(inherit)
      settings: CopyFcn=Stateflow.SLINSF.SimulinkMan.removeBlockPreDeleteFcn  PreDeleteFcn=Stateflow.SLINSF.SimulinkMan.unsafePredeleteFcn
  Constant : Constant
  Stop Simulation : Stop
  wires:
  Constant/1 -> Stop Simulation/1

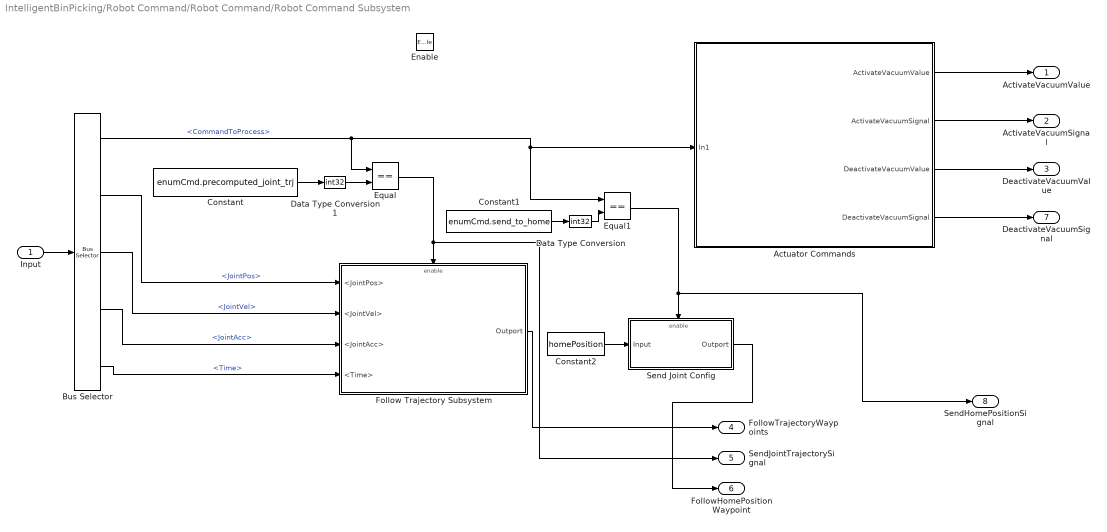
== system IntelligentBinPicking/Robot Command/Robot Command/Robot Command Subsystem ==
  Input : Inport
  Enable : EnablePort
  Actuator Commands : Subsystem  Variant=on
  Bus Selector : BusSelector  OutputSignals=CommandToProcess,JointTrajectory.JointPos,JointTrajectory.JointVel,JointTrajectory.JointAcc,JointTrajectory.Time
  Constant : Constant  Value=enumCmd.precomputed_joint_trj
  Constant1 : Constant  Value=enumCmd.send_to_home
  Constant2 : Constant  Value=homePosition
  Data Type Conversion : DataTypeConversion  OutDataTypeStr=int32  SaturateOnIntegerOverflow=off  RndMeth=Floor
  Data Type Conversion1 : DataTypeConversion  OutDataTypeStr=int32  SaturateOnIntegerOverflow=off  RndMeth=Floor
  Equal : RelationalOperator  Operator===  OutDataTypeStr=boolean  RndMeth=Simplest  InputSameDT=off
  Equal1 : RelationalOperator  Operator===  OutDataTypeStr=boolean  RndMeth=Simplest  InputSameDT=off
  Follow Trajectory Subsystem : Subsystem
  Send Joint Config : Subsystem  TreatAsAtomicUnit=on
  ActivateVacuumValue : Outport
  ActivateVacuumSignal : Outport  Port=2
  DeactivateVacuumValue : Outport  Port=3
  FollowTrajectoryWaypoints : Outport  Port=4
  SendJointTrajectorySignal : Outport  Port=5
  FollowHomePositionWaypoint : Outport  Port=6
  DeactivateVacuumSignal : Outport  Port=7
  SendHomePositionSignal : Outport  Port=8
  wires:
  Input/1 -> Bus Selector/1
  Bus Selector/3 -> Follow Trajectory Subsystem/2(<JointVel>)  "<JointVel>"
  Bus Selector/4 -> Follow Trajectory Subsystem/3(<JointAcc>)  "<JointAcc>"
  Bus Selector/5 -> Follow Trajectory Subsystem/4(<Time>)  "<Time>"
  Bus Selector/1 -> Actuator Commands/1(In1), Equal1/1, Equal/1  "<CommandToProcess>"
  Constant/1 -> Data Type Conversion1/1
  Equal/1 -> SendJointTrajectorySignal/1, Follow Trajectory Subsystem/Enable
  Bus Selector/2 -> Follow Trajectory Subsystem/1(<JointPos>)  "<JointPos>"
  Constant1/1 -> Data Type Conversion/1
  Equal1/1 -> SendHomePositionSignal/1, Send Joint Config/Enable
  Constant2/1 -> Send Joint Config/1(Input)
  Data Type Conversion/1 -> Equal1/2
  Data Type Conversion1/1 -> Equal/2
  Send Joint Config/1(Outport) -> FollowHomePositionWaypoint/1
  Follow Trajectory Subsystem/1(Outport) -> FollowTrajectoryWaypoints/1
  Actuator Commands/1(ActivateVacuumValue) -> ActivateVacuumValue/1
  Actuator Commands/2(ActivateVacuumSignal) -> ActivateVacuumSignal/1
  Actuator Commands/3(DeactivateVacuumValue) -> DeactivateVacuumValue/1
  Actuator Commands/4(DeactivateVacuumSignal) -> DeactivateVacuumSignal/1

== system IntelligentBinPicking/Robot Feedback/Motion Status/Gazebo ==
  Constant : Constant  Value=false
  Out1 : Outport
  wires:
  Constant/1 -> Out1/1

== system IntelligentBinPicking/Robot Feedback/Motion Status/Hardware ==
  MATLAB System : MATLABSystem  System=MotionStatusUR  ROSDeviceAddress=ROSDeviceAddress
      mask Type: MotionStatusUR
      mask Display:
      | disp('MotionStatusUR');
      | port_label('output',1,'success');
  NOT : Logic  Operator=NOT  AllPortsSameDT=off  OutDataTypeStr=boolean
  Out1 : Outport
  wires:
  MATLAB System/1 -> NOT/1
  NOT/1 -> Out1/1

== system IntelligentBinPicking/Robot Feedback/Motion Status/Sim3d ==
  Constant : Constant  Value=false
  Out1 : Outport
  wires:
  Constant/1 -> Out1/1

== system IntelligentBinPicking/Robot Command/Robot Command/Robot Command Subsystem/Actuator Commands ==
  In1 : Inport
  Gazebo : Subsystem  VariantControl=targetEnv == TargetEnvs.Gazebo
  Hardware : Subsystem  VariantControl=targetEnv == TargetEnvs.Hardware
  Sim3d : Subsystem  VariantControl=targetEnv == TargetEnvs.Sim3d
  ActivateVacuumValue : Outport
  ActivateVacuumSignal : Outport  Port=2
  DeactivateVacuumValue : Outport  Port=3
  DeactivateVacuumSignal : Outport  Port=4

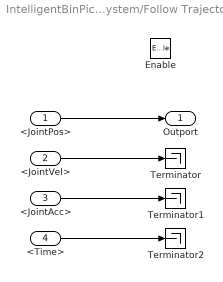
== system IntelligentBinPicking/Robot Command/Robot Command/Robot Command Subsystem/Follow Trajectory Subsystem ==
  <JointPos> : Inport
  <JointVel> : Inport  Port=2
  <JointAcc> : Inport  Port=3
  <Time> : Inport  Port=4
  Enable : EnablePort
  Terminator : Terminator
  Terminator1 : Terminator
  Terminator2 : Terminator
  Outport : Outport
  wires:
  <JointVel>/1 -> Terminator/1
  <JointAcc>/1 -> Terminator1/1
  <JointPos>/1 -> Outport/1
  <Time>/1 -> Terminator2/1

== system IntelligentBinPicking/Robot Command/Robot Command/Robot Command Subsystem/Send Joint Config ==
  Input : Inport
  Enable : EnablePort
  Outport : Outport
  wires:
  Input/1 -> Outport/1
